simulink model "test_tools"  (R2015b)
settings: Solver=FixedStepDiscrete  StartTime=0.0  StopTime=Inf  FixedStep=0.001  RelTol=1e-3
PostLoadFcn:
  | , if any(exist('dsrtsu_mdlpostloadfcn', 'file') == [2, 3, 6]), try dsrtsu_mdlpostloadfcn('Execute', bdroot); catch fprintf('Error in PostLoadFcn (dsrtsu_mdlpostloadfcn) for model "%s":\n %s\n', bdroot, lasterr); end, end,
libraries: tools x4
settings Model: DSRTSU_INTERNAL_RTI_VER=460  DSRTSU_INTERNAL_RTI_TYPE=rti1401  DSRTSU_INTERNAL_RTIFPGA=50  Creator=luis  LastModifiedBy=luis
settings SolverCC: AutoInsertRateTranBlk=on  InsertRTBMode=Always
settings OptimizationCC: BlockReduction=off  OptimizeBlockIOStorage=off  BufferReuse=off  GlobalBufferReuse=off  ExpressionFolding=off  LocalBlockOutputs=off
settings HardwareCC: ProdEndianess=BigEndian  ProdWordSize=32  ProdHWDeviceType=Generic->Custom  TargetIntDivRoundTo=Zero  TargetEndianess=BigEndian  TargetHWDeviceType=Generic->Custom
settings RTWCC: SystemTargetFile=rti1401.tlc  MakeCommand=make_rti  TemplateMakefile=rti1401.tmf  Description=dSPACE DS1401 Hardware Platform
settings STFCustomTargetCC: ParMdlRefBuildCompliant=on  ConcurrentExecutionCompliant=off  GeneratePreprocessorConditionals=Use local settings  MatFileLogging=on  CPPClassGenCompliant=off  SystemTargetFile=rti1401.tlc
settings GRTTargetCC: CompOptLevelCompliant=off  ConcurrentExecutionCompliant=off  CombineOutputUpdateFcns=off  CPPClassGenCompliant=off  GRTInterface=on  UseToolchainInfoCompliant=off  ExtModeMexFile=noextcomm

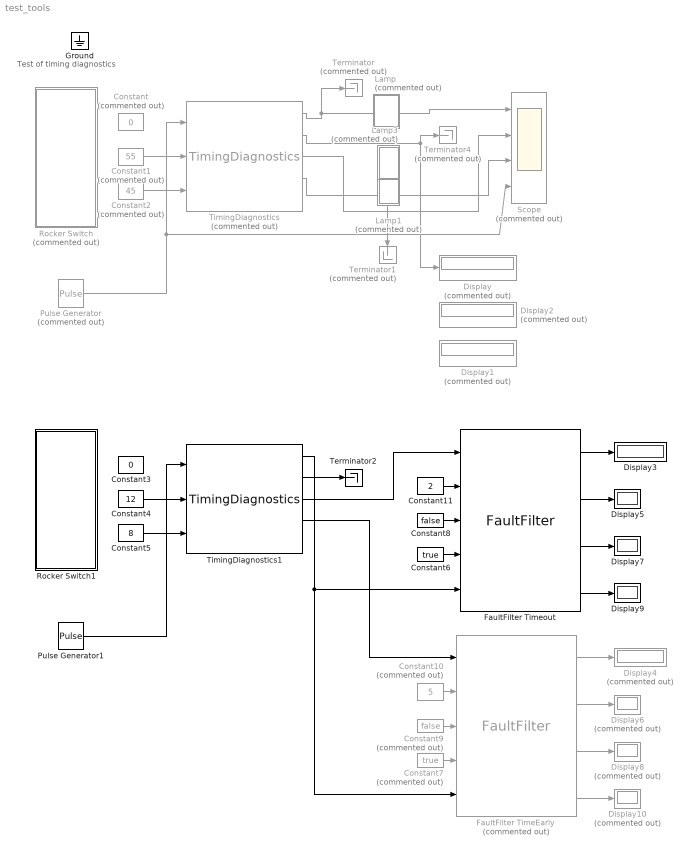
== system test_tools ==
  note: Test of timing diagnostics
  Constant : Constant  Commented=on  Value=0
  Constant1 : Constant  Commented=on  Value=55
  Constant10 : Constant  Commented=on  Value=5
  Constant11 : Constant  Value=2
  Constant2 : Constant  Commented=on  Value=45
  Constant3 : Constant  Value=0
  Constant4 : Constant  Value=12
  Constant5 : Constant  Value=8
  Constant6 : Constant  Value=true
  Constant7 : Constant  Commented=on  Value=true
  Constant8 : Constant  Value=false
  Constant9 : Constant  Commented=on  Value=false
  Display{,1..2,4,6,8,10} (7 alike) : Display  Commented=on
  Display{3,5,7,9} (4 alike) : Display
  FaultFilter TimeEarly : tools/FaultFilter  Commented=on
  FaultFilter Timeout : tools/FaultFilter
  Lamp : Subsystem  Commented=on  DialogController=hmiCreateDDGDialog  IsWebBlock=on  mask(MWDashboardBlock){webBlockId=ada42c60-518d-4ee7-a6cc-bb89c75a8cf9, webBlockType=lamp, ShowInLibBrowser=on, ShowInitialText=on, HMISrcModelName=test_tools}
      mask prompts: webBlockType "WebBlock Type"; HMISrcModelName "Source Model"
      mask Help: helpview([docroot '/mapfiles/simulink.map'], 'hmi_lamp')
      mask Display:
      | if strcmp(get_param(bdroot(gcb),'BlockDiagramType'), 'library')
      |     image([(matlabroot) '/toolbox/simulink/hmi/icons/Lamp.png']);
      | end
  Lamp1 : Subsystem  Commented=on  DialogController=hmiCreateDDGDialog  IsWebBlock=on  mask(MWDashboardBlock){webBlockId=325fee74-fc58-4102-b031-1dcf5c8417a6, webBlockType=lamp, ShowInLibBrowser=on, ShowInitialText=on, HMISrcModelName=test_tools}
      mask prompts: webBlockType "WebBlock Type"; HMISrcModelName "Source Model"
      mask Help: helpview([docroot '/mapfiles/simulink.map'], 'hmi_lamp')
      mask Display:
      | if strcmp(get_param(bdroot(gcb),'BlockDiagramType'), 'library')
      |     image([(matlabroot) '/toolbox/simulink/hmi/icons/Lamp.png']);
      | end
  Lamp3 : Subsystem  Commented=on  DialogController=hmiCreateDDGDialog  IsWebBlock=on  mask(MWDashboardBlock){webBlockId=b6e0b2c0-6f5c-4c4c-90e4-7dc0884d543e, webBlockType=lamp, ShowInLibBrowser=on, ShowInitialText=on, HMISrcModelName=test_tools}
      mask prompts: webBlockType "WebBlock Type"; HMISrcModelName "Source Model"
      mask Help: helpview([docroot '/mapfiles/simulink.map'], 'hmi_lamp')
      mask Display:
      | if strcmp(get_param(bdroot(gcb),'BlockDiagramType'), 'library')
      |     image([(matlabroot) '/toolbox/simulink/hmi/icons/Lamp.png']);
      | end
  Pulse Generator : DiscretePulseGenerator  Commented=on  Period=46  PhaseDelay=46  SampleTime=-1
  Pulse Generator1 : DiscretePulseGenerator  Period=15  SampleTime=-1
  Rocker Switch : Subsystem  Commented=on  DialogController=hmiCreateDDGDialog  IsWebBlock=on  mask(MWDashboardBlock){webBlockId=b0a97723-fc0e-4bed-842b-dfdeef123960, webBlockType=rockerswitch, ShowInLibBrowser=on, ShowInitialText=on, HMISrcModelName=test_tools}
      mask prompts: webBlockId "WebBlock Id"; webBlockType "WebBlock Type"; HMISrcModelName "Source Model"
      mask Help: helpview([docroot '/mapfiles/simulink.map'], 'hmi_rocker_switch')
      mask Display:
      | if strcmp(get_param(bdroot(gcb),'BlockDiagramType'), 'library')
      |     image([(matlabroot) '/toolbox/simulink/hmi/icons/RockerSwitch.png']);
      | end
  Rocker Switch1 : Subsystem  DialogController=hmiCreateDDGDialog  IsWebBlock=on  mask(MWDashboardBlock){webBlockId=a2a68395-64d0-4adc-8d56-22706fc50f37, webBlockType=rockerswitch, ShowInLibBrowser=on, ShowInitialText=on, HMISrcModelName=test_tools}
      mask prompts: webBlockId "WebBlock Id"; webBlockType "WebBlock Type"; HMISrcModelName "Source Model"
      mask Help: helpview([docroot '/mapfiles/simulink.map'], 'hmi_rocker_switch')
      mask Display:
      | if strcmp(get_param(bdroot(gcb),'BlockDiagramType'), 'library')
      |     image([(matlabroot) '/toolbox/simulink/hmi/icons/RockerSwitch.png']);
      | end
  Scope : Scope  Commented=on  NumInputPorts=4
  Terminator : Terminator  Commented=on
  Terminator1 : Terminator  Commented=on
  Terminator2 : Terminator
  Terminator4 : Terminator  Commented=on
  TimingDiagnostics : tools/TimingDiagnostics  Commented=on
  TimingDiagnostics1 : tools/TimingDiagnostics
  Ground : Ground  IOType=siggen
  wires:
  TimingDiagnostics/2 -> Terminator4/1, Display/1
  TimingDiagnostics/3 -> Scope/2
  TimingDiagnostics/4 -> Scope/3, Terminator1/1
  Constant1/1 -> TimingDiagnostics/2
  Constant2/1 -> TimingDiagnostics/3
  TimingDiagnostics/1 -> Terminator/1, Scope/1
  Pulse Generator/1 -> Scope/4, TimingDiagnostics/1
  Constant4/1 -> TimingDiagnostics1/2
  Constant5/1 -> TimingDiagnostics1/3
  Pulse Generator1/1 -> TimingDiagnostics1/1
  TimingDiagnostics1/2 -> Terminator2/1
  TimingDiagnostics1/3 -> FaultFilter Timeout/1
  TimingDiagnostics1/4 -> FaultFilter TimeEarly/1
  Constant6/1 -> FaultFilter Timeout/4
  Constant7/1 -> FaultFilter TimeEarly/4
  Constant8/1 -> FaultFilter Timeout/3
  Constant9/1 -> FaultFilter TimeEarly/3
  Constant10/1 -> FaultFilter TimeEarly/2
  Constant11/1 -> FaultFilter Timeout/2
  FaultFilter Timeout/1 -> Display3/1
  FaultFilter TimeEarly/1 -> Display4/1
  FaultFilter Timeout/2 -> Display5/1
  FaultFilter TimeEarly/2 -> Display6/1
  FaultFilter Timeout/3 -> Display7/1
  FaultFilter TimeEarly/3 -> Display8/1
  FaultFilter Timeout/4 -> Display9/1
  FaultFilter TimeEarly/4 -> Display10/1
  TimingDiagnostics1/1 -> FaultFilter Timeout/5, FaultFilter TimeEarly/5

== system test_tools/Lamp ==

== system test_tools/Lamp1 ==

== system test_tools/Lamp3 ==

== system test_tools/Rocker Switch ==

== system test_tools/Rocker Switch1 ==
